simulink model "zeroInitialSpeed"  (R2014b)
settings: Solver=ode23  StartTime=0.0  StopTime=5  MaxStep=0.01  RelTol=1e-3  AbsTol=1E-6
Description:
  | Bouncing Ball Model
  | 
  | This model calculates the trajectory, over time, of a ball thrown
  | upward with a velocity of 15 meters per second from a height of 10 m.
  | The model demonstrates the use of the 'ReinitDXDTwhenXreachesSaturation'
  | parameter in the Second-Order Integrator block to model this system.
  | This parameter, when set to 'on', forces a reinitialization of dx/dt
  | (velocity in the model) at the instant when x (position) reaches
  | saturation (i.e., when the ball hits the ground). The reinitialized value
  | is calculated by multiplying a coefficient of restitution times the ball
  | velocity, the instant before the ball hits the ground. The Memory block
  | in the calculation loop serves to capture the velocity of the ball just
  | before it hits the ground. The position of the ball is plotted in the
  | upper axis of the scope while the velocity of the ball is plotted in
  | the lower axis.
settings Model: Creator=The MathWorks Inc.  LastModifiedBy=geoHeil
settings DataIOCC: LimitDataPoints=off  MaxDataPoints=7500  SaveOutput=off  SignalLogging=off  DSMLogging=off  SaveTime=off
settings OptimizationCC: ExpressionDepthLimit=2147483647  EfficientFloat2IntCast=on
settings DebuggingCC: UnderspecifiedInitializationDetection=Classic  MergeDetectMultiDrivingBlocksExec=none  IgnoredZcDiagnostic=none  SolverPrmCheckMsg=none  FcnCallInpInsideContextMsg=EnableAllAsWarning  StateNameClashWarn=warning
settings HardwareCC: TargetBitPerLong=64  TargetBitPerPointer=64  TargetLongLongMode=on  TargetEndianess=LittleEndian  TargetWordSize=64  TargetHWDeviceType=MATLAB Host  ProdEqTarget=off
settings RTWCC: SystemTargetFile=rsim.tlc  TemplateMakefile=rsim_default_tmf  Description=Rapid Simulation Target  ProcessScript=rsim_make_rtw_hook
settings TargetCC: ParMdlRefBuildCompliant=on  ConcurrentExecutionCompliant=on  MatFileLogging=on  EnableShiftOperators=on

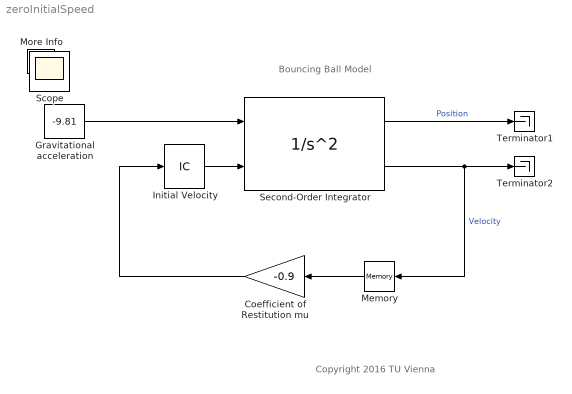
== system zeroInitialSpeed ==
  note: Copyright 2016 TU Vienna
  note: Bouncing Ball Model
  Coefficient of Restitution mu : Gain  Gain=-0.9
  Gravitational acceleration : Constant  Value=-9.81  OutDataTypeStr=double
  "Initial Velocity " : InitialCondition  Value=0
  Memory : Memory
  More Info : Subsystem
      settings: OpenFcn=showdemo(bdroot(gcs))
      mask Display: disp('?')
  Second-Order Integrator : SecondOrderIntegrator  ICX=10.0  LimitX=on  LowerLimitX=0.0  StateNameX='Position'  ICSourceDXDT=external  StateNameDXDT='Velocity'  ReinitDXDTwhenXreachesSaturation=on
  Terminator1 : Terminator
  Terminator2 : Terminator
  Scope : Scope  NumInputPorts=2
      settings: TimeRange=25  YMin=0~-30  YMax=25~20  MaxDataPoints=7500
  wires:
  Gravitational acceleration/1 -> Second-Order Integrator/1
  Second-Order Integrator/1 -> Terminator1/1  "Position"
  Second-Order Integrator/2 -> Memory/1, Terminator2/1  "Velocity"
  Memory/1 -> Coefficient of Restitution mu/1
  "Initial Velocity "/1 -> Second-Order Integrator/2
  Coefficient of Restitution mu/1 -> "Initial Velocity "/1

== system zeroInitialSpeed/More Info ==
